simulink model "untitled_mhi"  (Simulink 7.4)
settings: Solver=FixedStepDiscrete  StartTime=0.0  StopTime=inf  RelTol=1e-3
undefined symbols (not defined in the file): gray, jet, pause
libraries: simulink x3, vipsnks x3, dspstat3 x2, dspsrcs4 x1, vipsrcs x1, vipanalysis x1
settings Model: Creator=student  LastModifiedBy=student

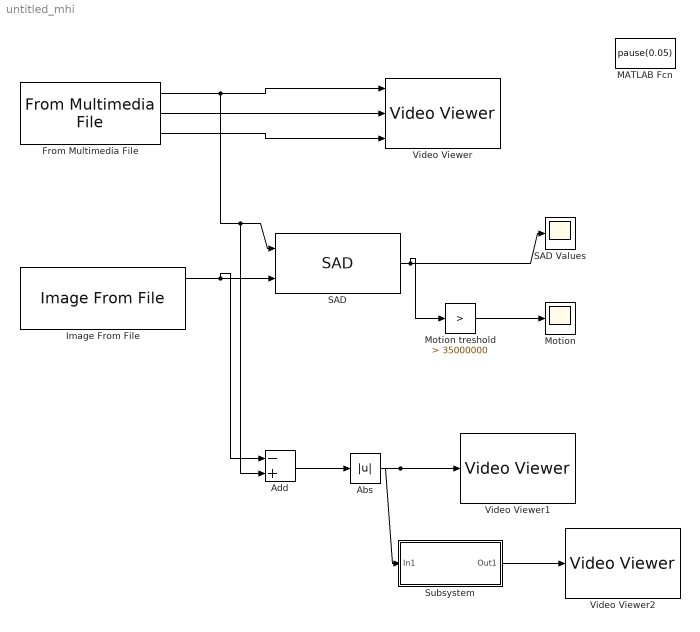
== system untitled_mhi ==
  Abs : Abs  OutDataTypeMode=int16  OutDataType=fixdt(1, 16)  OutScaling=2^0  OutDataTypeStr=int16
  Add : Sum  Inputs=-+  AccumDataTypeStr=int16  OutDataTypeMode=int16  OutDataType=fixdt(1, 16)  OutScaling=2^-10  OutDataTypeStr=int16
  From Multimedia File : dspsrcs4/From Multimedia File  DialogController=dspDDGCreate  DialogControllerArgs=DataTag0  inputFilename=D:\Multimodal\pn-0930\lab-3\motion1.avi  loop=on  numPlays=inf  outputStreams=Video only  videoDataType=int16  audioDataType=int16  inheritSampleTime=on  userDefinedSampleTime=1/30  noAudioOutput=off  isIntensityVideo=off  colorVideoFormat=Separate color signals  outputEOF=off  dataOrg=Column-major  audioFrameSize=1024
  Image From File : vipsrcs/Image From File  Tag=vipblks_nd  DialogController=vipDDGCreate  DialogControllerArgs=DataTag1  SystemSampleTime=-1  FileName=D:\Multimodal\pn-0930\lab-3\tlo0000.bmp  imagePorts=Separate color signals  Ts=inf  ImageDataType=int16  Signed=on  WordLength=16  sdImageDataType=uint(8)  FractionLengthMode=User-defined  FractionLength=15  OutPortLabels=R|G|B
  MATLAB Fcn : MATLABFcn  MATLABFcn=pause(0.05)  OutputDimensions=0
  Motion : Scope
      settings: YMin=0  YMax=1
  Motion treshold : simulink/Logic and Bit Operations/Compare To Constant  SystemSampleTime=-1  relop=>  const=35000000  LogicOutDataTypeMode=uint8
  SAD : vipanalysis/SAD  DialogController=vipDDGCreate  DialogControllerArgs=DataTag2  output=SAD values  method=Exhaustive  roi=off  invalidROI=Ignore  nearbyPel=off  nearbySize=3  outputMode=Binary point scaling  outputWordLength=32  outputFracLength=0  accumMode=Binary point scaling  accumWordLength=32  accumFracLength=0  roundingMode=Floor  overflowMode=off
  SAD Values : Scope
      settings: YMin=2.5e+007  YMax=8e+007
  Subsystem : Subsystem
  Video Viewer : vipsnks/Video Viewer  DialogControllerArgs=DataTag6  inputType=Obsolete7b  imagePorts=Separate color signals  useColorMap=off  colormapValue=gray(256)  specRange=off  minInputVal=0  maxInputVal=255  FigPos=[895 985 410 300]  AxisZoom=on  trueSizedOnce=off  OpenAtMdlStart=on
  Video Viewer1 : vipsnks/Video Viewer  DialogControllerArgs=DataTag8  inputType=Obsolete7b  imagePorts=One multidimensional signal  useColorMap=off  colormapValue=gray(256)  specRange=off  minInputVal=0  maxInputVal=255  FigPos=[37 951 410 300]  AxisZoom=on  trueSizedOnce=off  OpenAtMdlStart=on
  Video Viewer2 : vipsnks/Video Viewer  DialogControllerArgs=DataTag10  inputType=Obsolete7b  imagePorts=One multidimensional signal  useColorMap=on  colormapValue=jet(256)  specRange=on  minInputVal=0  maxInputVal=6  FigPos=[38 530 410 300]  AxisZoom=on  trueSizedOnce=off  OpenAtMdlStart=on
  wires:
  From Multimedia File/1 -> Video Viewer/1, SAD/1, Add/2
  From Multimedia File/2 -> Video Viewer/2
  From Multimedia File/3 -> Video Viewer/3
  Image From File/1 -> SAD/2, Add/1
  SAD/1 -> Motion treshold/1, SAD Values/1
  Motion treshold/1 -> Motion/1
  Add/1 -> Abs/1
  Abs/1 -> Video Viewer1/1, Subsystem/1(In1)
  Subsystem/1(Out1) -> Video Viewer2/1

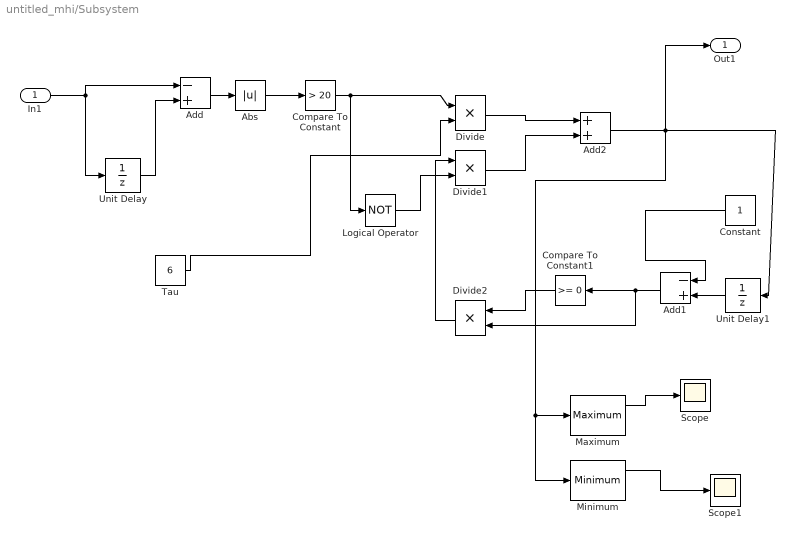
== system untitled_mhi/Subsystem ==
  In1 : Inport  OutDataType=fixdt(1, 16)  OutScaling=2^0
  Abs : Abs  OutDataTypeMode=uint8  OutDataType=fixdt(1, 16)  OutScaling=2^0  OutDataTypeStr=uint8
  Add : Sum  Inputs=-+  OutDataTypeMode=int16  OutDataType=fixdt(1, 16)  OutScaling=2^-10  OutDataTypeStr=int16
  Add1 : Sum  Inputs=-+  OutDataType=fixdt(1, 16)  OutScaling=2^-10
  Add2 : Sum  OutDataType=fixdt(1, 16)  OutScaling=2^-10
  Compare To Constant : simulink/Logic and Bit Operations/Compare To Constant  SystemSampleTime=-1  relop=>  const=20  LogicOutDataTypeMode=boolean
  Compare To Constant1 : simulink/Logic and Bit Operations/Compare To Constant  SystemSampleTime=-1  relop=>=  const=0  LogicOutDataTypeMode=uint8
  Constant : Constant  OutDataType=fixdt(1, 16)  OutScaling=2^0
  Divide : Product  Inputs=**  OutDataType=fixdt(1, 16)  OutScaling=2^-10
  Divide1 : Product  Inputs=**  OutDataType=fixdt(1, 16)  OutScaling=2^-10
  Divide2 : Product  Inputs=**  OutDataType=fixdt(1, 16)  OutScaling=2^-10
  Logical Operator : Logic  Operator=NOT  AllPortsSameDT=off  OutDataTypeMode=boolean  LogicDataType=fixdt(0, 8)  OutDataTypeStr=boolean
  Maximum : dspstat3/Maximum  DialogController=dspDDGCreate  DialogControllerArgs=DataTag3  fcn=Value and Index  reset=None  indexBase=Zero  operateOver=Entire input  Dimension=1  colComp=on  operation=maximum  roiEnable=off  roiType=Rectangles  roiPortion=Entire ROI  roiOutput=Individual statistics for each ROI  roiFlag=off  accumDataTypeStr=Inherit: Same as product output  accumLastDataTypeStr=Inherit: Same as product output  roundingMode=Floor  overflowMode=off
  Minimum : dspstat3/Minimum  DialogController=dspDDGCreate  DialogControllerArgs=DataTag4  fcn=Value and Index  reset=None  indexBase=Zero  operateOver=Entire input  Dimension=1  colComp=on  operation=minimum  roiEnable=off  roiType=Rectangles  roiPortion=Entire ROI  roiOutput=Individual statistics for each ROI  roiFlag=off  accumDataTypeStr=Inherit: Same as product output  accumLastDataTypeStr=Inherit: Same as product output  roundingMode=Floor  overflowMode=off
  Scope : Scope
      settings: SaveName=ScopeData2
  Scope1 : Scope
      settings: SaveName=ScopeData3
  Tau : Constant  Value=6  OutDataType=fixdt(1, 16)  OutScaling=2^0
  Unit Delay : UnitDelay  SampleTime=-1
  Unit Delay1 : UnitDelay  SampleTime=-1
  Out1 : Outport  OutDataType=fixdt(1, 16)  OutScaling=2^0
  wires:
  In1/1 -> Unit Delay/1, Add/1
  Unit Delay/1 -> Add/2
  Add/1 -> Abs/1
  Abs/1 -> Compare To Constant/1
  Compare To Constant/1 -> Divide/1, Logical Operator/1
  Logical Operator/1 -> Divide1/2
  Divide2/1 -> Divide1/1
  Compare To Constant1/1 -> Divide2/1
  Add1/1 -> Compare To Constant1/1, Divide2/2
  Divide/1 -> Add2/1
  Divide1/1 -> Add2/2
  Add2/1 -> Unit Delay1/1, Out1/1, Maximum/1, Minimum/1
  Unit Delay1/1 -> Add1/2
  Constant/1 -> Add1/1
  Tau/1 -> Divide/2
  Maximum/1 -> Scope/1
  Minimum/1 -> Scope1/1
